simulink model "switch_controller_eMPC"  (R2020a)
settings: Solver=VariableStepAuto  StartTime=0.0  StopTime=10.0  RelTol=1e-3
undefined symbols (not defined in the file): G, us, xs
libraries: powerlib x11, eeLuenbergerObserver x2, powerlib_meascontrol x1, eeGeneralControl x1
settings Model: Creator=Slash  LastModifiedBy=Slash

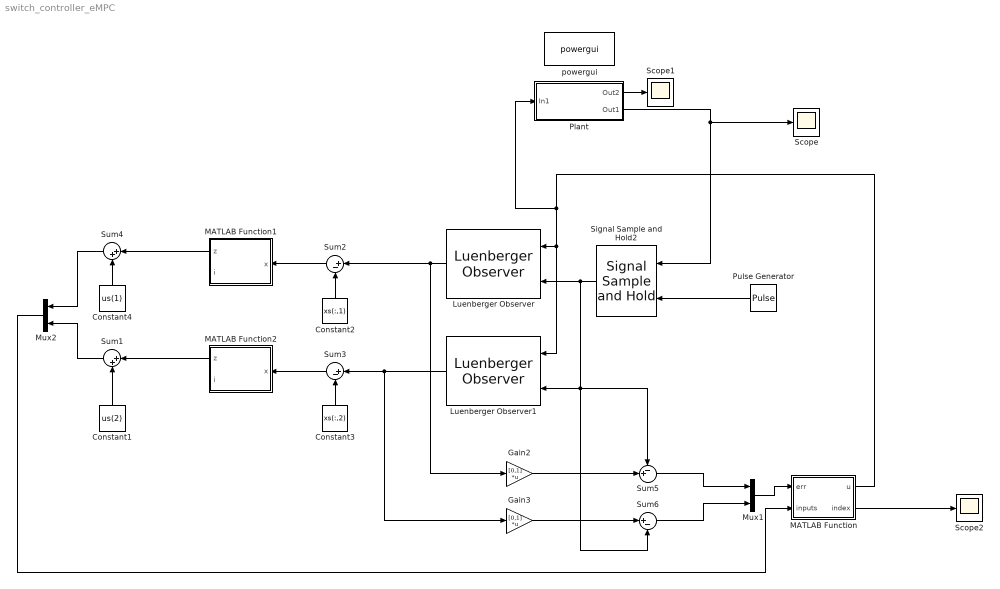
== system switch_controller_eMPC ==
  Constant1 : Constant  Value=us(2)
  Constant2 : Constant  Value=xs(:,1)
  Constant3 : Constant  Value=xs(:,2)
  Constant4 : Constant  Value=us(1)
  Gain2 : Gain  Gain=[0,1]  Multiplication=Matrix(K*u)
  Gain3 : Gain  Gain=[0,1]  Multiplication=Matrix(K*u)
  Luenberger Observer : eeLuenbergerObserver/Luenberger Observer  StateSpaceType=Discrete-time  Ad=G(:,:,1,1).A  Bd=G(:,:,1,1).B  Cd=[0,1]  Dd=0  A=1  B=1  C=1  D=1  ObserverDesign=Desired eigenvalues  Ld=[0;0]  DesiredEigenvalues=[0.2,0.21]  x0=[0,0]  Tsd=0.1  Ts=0.001
      settings: SourceProductBaseCode=PS
  Luenberger Observer1 : eeLuenbergerObserver/Luenberger Observer  StateSpaceType=Discrete-time  Ad=G(:,:,2,1).A  Bd=G(:,:,2,1).B  Cd=[0,1]  Dd=0  A=1  B=1  C=1  D=1  ObserverDesign=Desired eigenvalues  Ld=[0;0]  DesiredEigenvalues=[0.2,0.21]  x0=[0,0]  Tsd=0.1  Ts=0.001
      settings: SourceProductBaseCode=PS
  MATLAB Function : MATLAB Function  TreatAsAtomicUnit=on
  MATLAB Function1 : MATLAB Function  TreatAsAtomicUnit=on
  MATLAB Function2 : MATLAB Function  TreatAsAtomicUnit=on
  Mux1 : Mux  Inputs=2
  Mux2 : Mux  Inputs=2
  Plant : Subsystem
  Pulse Generator : DiscretePulseGenerator  PulseType=Time based  Period=0.001
  Scope : Scope
  Scope1 : Scope
  Scope2 : Scope
  Signal Sample and Hold2 : eeGeneralControl/Signal Sample and Hold  LabelModeActiveChoice=Discrete  x0=0  Ts=0.001
      settings: SourceProductBaseCode=PS
  Sum1 : Sum  Inputs=|++
  Sum2 : Sum  Inputs=|+-
  Sum3 : Sum  Inputs=|+-
  Sum4 : Sum  Inputs=|++
  Sum5 : Sum  Inputs=-+|
  Sum6 : Sum  Inputs=|+-
  powergui : powerlib/powergui  Priority=1  SimulationMode=Continuous  SampleTime=50e-6  frequency=60  Iterations=50  frequencyindice=0  Pbase=100e6  ErrMax=1e-4  UnitsV=kV  UnitsW=MW  buscounter=0  FunctionMessages=off  echomessages=off  EnableUseOfTLC=off  CurrentSourceSwitches=off  DisableSnubberDevices=off  DisableRonSwitches=off  DisableVfSwitches=off  DisplayEquations=off  AutomaticDiscreteSolvers=off  SolverType=Tustin/Backward Euler (TBE)  Interpol=off  ExternalGateDelay=off  methode=off  Ts=100  x0status=blocks  SPID=on  SwTol=0  HookPort=off  NonlinearTolerance=1e-4  nMaxIteration=100  ContinueOnMaxIteration=off  RestoreLinks=warning  ResistiveCurrentMeasurement=off  Frange=[0:2:500]  Ylog=off  Xlog=on  ShowGrid=off  save=off  variable=ZData  structure=0  ZoomFFT=off  StartTime=0.0  cycles=1  DisplayStyle=1  fundamental=60  FreqAxis=off  MaxFrequency=1000  frequencyindicesteady=1  RmsSteady=1  display=off
  wires:
  MATLAB Function/2(index) -> Scope2/1
  Constant1/1 -> Sum1/2
  Sum1/1 -> Mux2/2
  Plant/1(Out2) -> Scope1/1
  Sum3/1 -> MATLAB Function2/1(x)
  Mux1/1 -> MATLAB Function/1(err)
  Constant3/1 -> Sum3/2
  Constant4/1 -> Sum4/2
  Gain2/1 -> Sum5/2
  MATLAB Function1/1(z) -> Sum4/1
  Signal Sample and Hold2/1 -> Sum6/2, Luenberger Observer1/2, Sum5/1, Luenberger Observer/2
  Sum4/1 -> Mux2/1
  Gain3/1 -> Sum6/1
  Sum5/1 -> Mux1/1
  Sum6/1 -> Mux1/2
  Constant2/1 -> Sum2/2
  Luenberger Observer/1 -> Gain2/1, Sum2/1
  Plant/2(Out1) -> Signal Sample and Hold2/1, Scope/1
  Luenberger Observer1/1 -> Gain3/1, Sum3/1
  MATLAB Function/1(u) -> Plant/1(In1), Luenberger Observer/1, Luenberger Observer1/1
  Pulse Generator/1 -> Signal Sample and Hold2/2
  Mux2/1 -> MATLAB Function/2(inputs)
  Sum2/1 -> MATLAB Function1/1(x)
  MATLAB Function2/1(z) -> Sum1/1

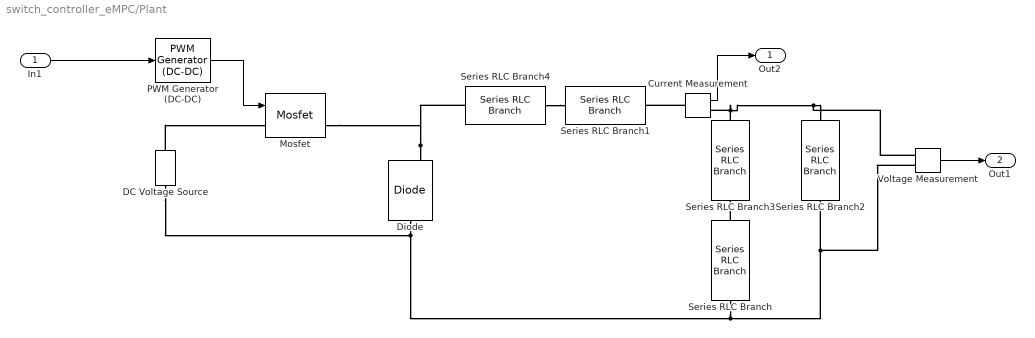
== system switch_controller_eMPC/Plant ==
  In1 : Inport
  Current Measurement : powerlib/Measurements/Current Measurement  PhasorSimulation=off  OutputType=Complex  PSBequivalent=0
  DC Voltage Source : powerlib/Electrical Sources/DC Voltage Source  Amplitude=15  Measurements=None
  Diode : powerlib/Power Electronics/Diode  Ron=0.001  Lon=0  Vf=0.1  IC=0  UseSnubber=0  Rs=500  Cs=250e-9  Measurements=on
  Mosfet : powerlib/Power Electronics/Mosfet  Ron=0.05  Lon=0  Rd=0.01  Vfd=0  IC=0  Rs=1e5  Cs=inf  Measurements=on
  PWM Generator (DC-DC) : powerlib_meascontrol/Pulse & Signal Generators/PWM Generator (DC-DC)  Fsw=20000  Ts=0
  Series RLC Branch : powerlib/Elements/Series RLC Branch  LConnTagsString=__new0  RConnTagsString=__new0  BranchType=C  Resistance=1  Inductance=1e-3  SetiL0=off  InitialCurrent=0  Capacitance=56e-6  Setx0=off  InitialVoltage=0  Measurements=None
  Series RLC Branch1 : powerlib/Elements/Series RLC Branch  LConnTagsString=__new0  RConnTagsString=__new0  BranchType=L  Resistance=1  Inductance=10e-3  SetiL0=off  InitialCurrent=0  Capacitance=1e-6  Setx0=off  InitialVoltage=0  Measurements=None
  Series RLC Branch2 : powerlib/Elements/Series RLC Branch  LConnTagsString=__new0  RConnTagsString=__new0  BranchType=R  Resistance=100  Inductance=1e-3  SetiL0=off  InitialCurrent=0  Capacitance=1e-6  Setx0=off  InitialVoltage=0  Measurements=None
  Series RLC Branch3 : powerlib/Elements/Series RLC Branch  LConnTagsString=__new0  RConnTagsString=__new0  BranchType=R  Resistance=0.33  Inductance=1e-3  SetiL0=off  InitialCurrent=0  Capacitance=1e-6  Setx0=off  InitialVoltage=0  Measurements=None
  Series RLC Branch4 : powerlib/Elements/Series RLC Branch  LConnTagsString=__new0  RConnTagsString=__new0  BranchType=R  Resistance=1.6  Inductance=1e-3  SetiL0=off  InitialCurrent=0  Capacitance=1e-6  Setx0=off  InitialVoltage=0  Measurements=None
  Voltage Measurement : powerlib/Measurements/Voltage Measurement  PhasorSimulation=off  OutputType=Complex  PSBequivalent=0
  Out2 : Outport
  Out1 : Outport  Port=2
  wires:
  Voltage Measurement/1 -> Out1/1
  PWM Generator (DC-DC)/1 -> Mosfet/1
  In1/1 -> PWM Generator (DC-DC)/1
  Current Measurement/1 -> Out2/1
  connections:
  Diode/LConn1 -- DC Voltage Source/LConn1 -- Voltage Measurement/LConn2 -- Series RLC Branch2/RConn1 -- Series RLC Branch/RConn1
  Diode/RConn1 -- Series RLC Branch4/RConn1 -- Mosfet/RConn1
  Series RLC Branch3/LConn1 -- Current Measurement/RConn1 -- Series RLC Branch2/LConn1 -- Voltage Measurement/LConn1
  Series RLC Branch/LConn1 -- Series RLC Branch3/RConn1
  DC Voltage Source/RConn1 -- Mosfet/LConn1
  Series RLC Branch4/LConn1 -- Series RLC Branch1/LConn1
  Current Measurement/LConn1 -- Series RLC Branch1/RConn1

== matlab function switch_controller_eMPC/MATLAB Function1 ==
  settings: updateMethod=DISCRETE  sampleTime=0.001
  data: x input size=[2,1]; z output size=[1,1] [0..1]; i output
function [z,i] = exp_sol_100(x) %#codegen
%Evaluate function "primal" with tiebreak "obj"
% 
%  [value, region] = exp_sol_100(x)
%
%See "help PolyUnion/toMatlab" for more information.
x=x(:);xh=[x;-1];
if numel(x)~=2,error('The input vector must have 2 elements.');end
nx=2;nz=1;
H=[-1 0 0.05;0.995484759334458 0.094921514593991 0.119230377256846;0 -1 5;0.999456236344815 -0.0329731956512758 0.543916341112487;1 0 0.45;-1 0 0.05;0.995535067130876 0.0943924261406664 0.267817809440488;0.961311217383224 -0.275464595425953 1.3292574162606;-0.995484759334458 -0.094921514593991 -0.119230377256846;1 0 0.45;-0.961311217383224 0.275464595425953 -1.3292574162606;0 -1 5;-0.999456236344815 0.0329731956512758 -0.543916341112487;1 0 0.45;0 1 5;-1 0 0.05;0.995535067130877 0.0943924261406665 0.452285636184273;-0.995535067130877 -0.0943924261406663 -0.267817809440489;1 0 0.45;0 1 5;0.995535067130877 0.0943924261406665 0.642718821678027;-0.995535067130877 -0.0943924261406665 -0.452285636184273];
ni=[1;5;10;14;19;23];
fF=[-0.618391731398726 0.0204014451129071;-0.20781815132297 0.0595504784935119;0 0;-0.20781815132297 0.0595504784935119;-0.20781815132297 0.0595504784935119];
fg=[4.9960036108132e-16;-0.0491748792586778;-0.336536364160089;-0.0491748792586778;-0.0491748792586778];
tH=[135.682534103827 3.33425643971433;3.33425643971433 1.31775701387808;196.359761655315 9.11995459987719;9.11995459987719 1.86943520603192;273.33090557106 -1.20691957022027;-1.20691957022027 1.46757556482341;236.682637919419 12.9431992501214;12.9431992501214 2.23193909984848;263.178518785315 15.4554266544999;15.4554266544999 2.47013788113278];
tF=[-3.57523017875033e-15 -3.43343955629705e-16;-14.5347654276499 -1.38591970969329;-149.819863733824 4.9427273548359;-36.2300019852435 -3.44297031692994;-60.3049074895399 -5.72565107292491];
tg=[3.73286533643419e-28;0.870422951747174;40.7669036145563;3.78863795088998;9.25742268364088];
tb=[];
for i=1:5,
if all(H(ni(i):ni(i+1)-1,:)*xh<=1e-08);
tv=tF(i,:)*x+tg(i);
tv=tv+x'*tH((i-1)*nx+1:i*nx,:)*x;
tb=[tb;i,tv];
end
end
if ~isempty(tb)
[~,j]=min(tb(:,end));
i=tb(j,1);
z=fF((i-1)*nz+1:i*nz,:)*x+fg((i-1)*nz+1:i*nz);
return
end
i=0;z=NaN(1,1);
end

== matlab function switch_controller_eMPC/MATLAB Function ==
  data: err input size=2; u output size=1; inputs input size=2; index output
function [u,index] = fcn(err, inputs)
    err = err.^2;
    [~,index]=min(err);
    u = inputs(index);
end

== matlab function switch_controller_eMPC/MATLAB Function2 ==
  settings: updateMethod=DISCRETE  sampleTime=0.001
  data: x input size=[2,1]; z output size=[1,1] [0..1]; i output
function [z,i] = exp_sol_18(x) %#codegen
%Evaluate function "primal" with tiebreak "obj"
% 
%  [value, region] = exp_sol_18(x)
%
%See "help PolyUnion/toMatlab" for more information.
x=x(:);xh=[x;-1];
if numel(x)~=2,error('The input vector must have 2 elements.');end
nx=2;nz=1;
H=[1 0 0.222222222222222;0 1 5;-1 0 0.277777777777778;0 -1 5];
ni=[1;5];
fF=[-0.529982214636897 0.0250510149313122];
fg=0;
tH=[114.417357205858 0.936120031293399;0.936120031293399 1.06440493495907];
tF=[1.4716723152044e-16 1.30456018054158e-17];
tg=1.74783280394215e-28;
tb=[];
for i=1:1,
if all(H(ni(i):ni(i+1)-1,:)*xh<=1e-08);
tv=tF(i,:)*x+tg(i);
tv=tv+x'*tH((i-1)*nx+1:i*nx,:)*x;
tb=[tb;i,tv];
end
end
if ~isempty(tb)
[~,j]=min(tb(:,end));
i=tb(j,1);
z=fF((i-1)*nz+1:i*nz,:)*x+fg((i-1)*nz+1:i*nz);
return
end
i=0;z=NaN(1,1);
end
